simulink model "AvanzaBaldosa"  (R2023b)
settings: Solver=FixedStepAuto  StartTime=0.0  StopTime=inf  FixedStep=0.01  RelTol=1e-3  EnableMultiTasking=on
settings Model: ExtModeTrigDuration=2  Creator=Usuario  LastModifiedBy=Usuario
settings OptimizationCC: EnhancedBackFolding=on  PassReuseOutputArgsAs=Individual arguments  ZeroExternalMemoryAtStartup=off  ZeroInternalMemoryAtStartup=off  MaxStackSize=64  OptimizeBlockOrder=speed  DifferentSizesBufferReuse=on  OptimizationCustomize=off  EfficientTunableParamExpr=on
settings DebuggingCC: ParameterTunabilityLossMsg=error
settings HardwareCC: ProdBitPerInt=16  ProdBitPerPointer=16  ProdBitPerSizeT=16  ProdBitPerPtrDiffT=16  ProdLargestAtomicFloat=None  ProdWordSize=8  ProdHWDeviceType=Atmel->AVR  UseEmbeddedCoderFeatures=off  UseSimulinkCoderFeatures=off
settings SFSimCC: MATLABDynamicMemAlloc=off
settings RTWCC: Description=Embedded Coder  SystemTargetFile=ert.tlc  HardwareBoard=Arduino Mega 2560  TemplateMakefile=ert_default_tmf  Toolchain=Arduino AVR  BuildConfiguration=Faster Runs
settings CodeAppCC: ForceParamTrailComments=on  IgnoreCustomStorageClasses=off  OperatorAnnotations=on  SimulinkDataObjDesc=on  SFDataObjDesc=on  InsertBlockDesc=on
settings ERTTargetCC: SupportContinuousTime=on  SupportNonInlinedSFcns=on  SupportVariableSizeSignals=on  ExtModeTransport=3  ExtModeStaticAlloc=on  ExtModeAutomaticAllocSize=off  ExtModeStaticAllocSize=2048  ExtModeMexFile=ext_xcp  ExtModeIntrfLevel=Level2 - Open

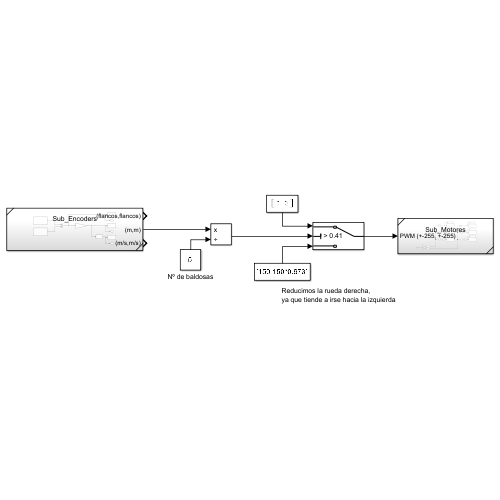
[thumbnail: Simulink's stored preview of the top-level diagram]
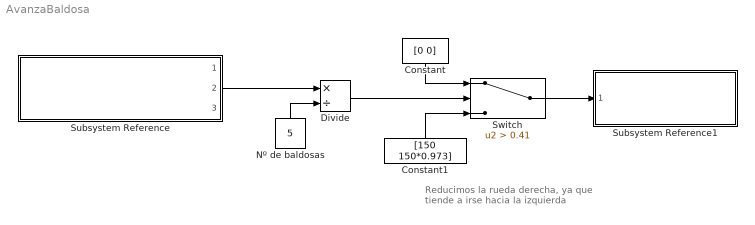
== system AvanzaBaldosa ==
  note: Reducimos la rueda derecha,
      | ya que tiende a irse hacia la izquierda
  Constant : Constant  Value=[0 0]
  Constant1 : Constant  Value=[150 150*0.973]
  Divide : Product  Inputs=*/
  Nº de baldosas : Constant  Value=5
  Subsystem Reference : Subsystem  ReferencedSubsystem=Sub_Encoders
  Subsystem Reference1 : Subsystem  ReferencedSubsystem=Sub_Motores
  Switch : Switch  Criteria=u2 > Threshold  Threshold=0.41  SaturateOnIntegerOverflow=off  InputSameDT=off
  wires:
  Constant/1 -> Switch/1
  Subsystem Reference/2 -> Divide/1
  Divide/1 -> Switch/2
  Nº de baldosas/1 -> Divide/2
  Constant1/1 -> Switch/3
  Switch/1 -> Subsystem Reference1/1
